simulink model "ISEmizgenj1"  (R2015a)
settings: Solver=ode45  StartTime=0.0  StopTime=10.0  RelTol=1e-3
undefined symbols (not defined in the file or in its folder): Kimiz2, Kpmiz2
settings Model: Creator=PC  LastModifiedBy=PC

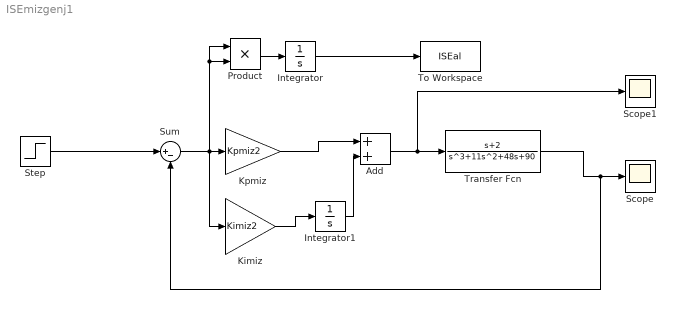
== system ISEmizgenj1 ==
  Add : Sum
  Integrator : Integrator
  Integrator1 : Integrator
  Kimiz : Gain  Gain=Kimiz2
  Kpmiz : Gain  Gain=Kpmiz2
  Product : Product
  Scope : Scope
  Scope1 : Scope
  Step : Step  SampleTime=0
  Sum : Sum  Inputs=|+-
  To Workspace : ToWorkspace  VariableName=ISEal  SampleTime=-1
  Transfer Fcn : TransferFcn  Numerator=[1 2]  Denominator=[1 11 48 90]
  wires:
  Sum/1 -> Product/2, Product/1, Kpmiz/1, Kimiz/1
  Step/1 -> Sum/1
  Product/1 -> Integrator/1
  Integrator/1 -> To Workspace/1
  Kimiz/1 -> Integrator1/1
  Integrator1/1 -> Add/2
  Kpmiz/1 -> Add/1
  Add/1 -> Scope1/1, Transfer Fcn/1
  Transfer Fcn/1 -> Sum/2, Scope/1
